simulink model "ROB599_HW5_P2D"  (R2023b)
settings: Solver=VariableStepAuto  StartTime=0.0  StopTime=10.0  RelTol=1e-3
libraries: cstblocks x2, simulink x1
settings Model: Creator=anatoliikalinin  LastModifiedBy=anatoliikalinin

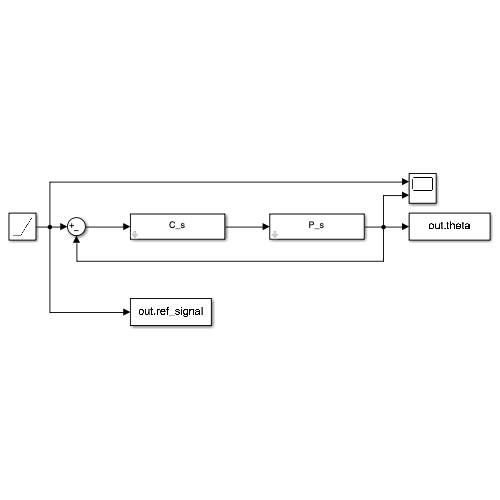
[thumbnail: Simulink's stored preview of the top-level diagram]
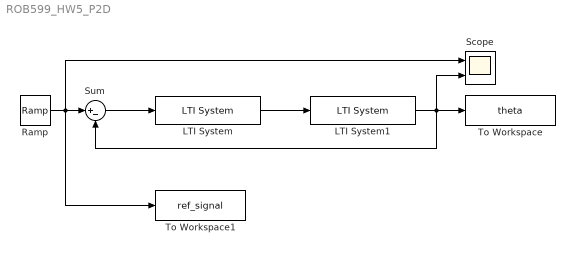
== system ROB599_HW5_P2D ==
  LTI System : cstblocks/LTI System  sys=C_s  IC=[]
  LTI System1 : cstblocks/LTI System  sys=P_s  IC=[]
  Ramp : simulink/Sources/Ramp  slope=1  start=0  InitialOutput=0
  Scope : Scope  NumInputPorts=2
  Sum : Sum  Inputs=|+-
  To Workspace : ToWorkspace  VariableName=theta  SaveFormat=Timeseries  SampleTime=-1
  To Workspace1 : ToWorkspace  VariableName=ref_signal  SaveFormat=Timeseries  SampleTime=-1
  wires:
  Sum/1 -> LTI System/1
  LTI System/1 -> LTI System1/1
  LTI System1/1 -> Scope/2, To Workspace/1, Sum/2
  Ramp/1 -> To Workspace1/1, Scope/1, Sum/1
